simulink library "GTPR_Library"  (R2021a)
settings: Solver=VariableStepAuto  StartTime=0.0  StopTime=10.0  RelTol=1e-3
values from neighbouring files (symbols this model uses):
  aA = 0.5    [SimMechanics_GTPR_OpenLoop_CircularMotion_VS_ClosedLoop.m]
  aB = 0.5    [SimMechanics_GTPR_OpenLoop_CircularMotion_VS_ClosedLoop.m]
  aC = 0.5    [SimMechanics_GTPR_OpenLoop_CircularMotion_VS_ClosedLoop.m]
  alphaAB = deg2rad(120)    [SimMechanics_GTPR_OpenLoop_CircularMotion_VS_ClosedLoop.m]
  alphaAC = deg2rad(240)    [SimMechanics_GTPR_OpenLoop_CircularMotion_VS_ClosedLoop.m]
  eA = 0.28    [SimMechanics_GTPR_OpenLoop_CircularMotion_VS_ClosedLoop.m]
  eB = 0.28    [SimMechanics_GTPR_OpenLoop_CircularMotion_VS_ClosedLoop.m]
  eC = 0.28    [SimMechanics_GTPR_OpenLoop_CircularMotion_VS_ClosedLoop.m]
  g = -9.81    [SimMechanics_GTPR_OpenLoop_CircularMotion_VS_ClosedLoop.m]
  ILA = zeros(3)    [SimMechanics_GTPR_OpenLoop_CircularMotion_VS_ClosedLoop.m]
  IlA = zeros(3)    [SimMechanics_GTPR_OpenLoop_CircularMotion_VS_ClosedLoop.m]
  ILB = zeros(3)    [SimMechanics_GTPR_OpenLoop_CircularMotion_VS_ClosedLoop.m]
  IlB = zeros(3)    [SimMechanics_GTPR_OpenLoop_CircularMotion_VS_ClosedLoop.m]
  ILC = zeros(3)    [SimMechanics_GTPR_OpenLoop_CircularMotion_VS_ClosedLoop.m]
  IlC = zeros(3)    [SimMechanics_GTPR_OpenLoop_CircularMotion_VS_ClosedLoop.m]
  LA = 0.57    [SimMechanics_GTPR_OpenLoop_CircularMotion_VS_ClosedLoop.m]
  lA = 0.9    [SimMechanics_GTPR_OpenLoop_CircularMotion_VS_ClosedLoop.m]
  LB = 0.57    [SimMechanics_GTPR_OpenLoop_CircularMotion_VS_ClosedLoop.m]
  lB = 0.9    [SimMechanics_GTPR_OpenLoop_CircularMotion_VS_ClosedLoop.m]
  LC = 0.57    [SimMechanics_GTPR_OpenLoop_CircularMotion_VS_ClosedLoop.m]
  lC = 0.9    [SimMechanics_GTPR_OpenLoop_CircularMotion_VS_ClosedLoop.m]
  m_unaccounted = 1e-16    [SimMechanics_GTPR_OpenLoop_CircularMotion_VS_ClosedLoop.m]
  mLA = density_upperArm*VLA    (= 1.4415197891)    [SimMechanics_GTPR_OpenLoop_CircularMotion_VS_ClosedLoop.m]
  mlA = density_LowerArm*VlA    (= 0.190851753706)    [SimMechanics_GTPR_OpenLoop_CircularMotion_VS_ClosedLoop.m]
  mLB = density_upperArm*VLB    (= 1.4415197891)    [SimMechanics_GTPR_OpenLoop_CircularMotion_VS_ClosedLoop.m]
  mlB = density_LowerArm*VlB    (= 0.190851753706)    [SimMechanics_GTPR_OpenLoop_CircularMotion_VS_ClosedLoop.m]
  mLC = density_upperArm*VLC    (= 1.4415197891)    [SimMechanics_GTPR_OpenLoop_CircularMotion_VS_ClosedLoop.m]
  mlC = density_LowerArm*VlC    (= 0.190851753706)    [SimMechanics_GTPR_OpenLoop_CircularMotion_VS_ClosedLoop.m]
  mTCP = density_workTriangle * VTCP    [SimMechanics_GTPR_OpenLoop_CircularMotion_VS_ClosedLoop.m]
undefined symbols (not defined in the file or in its folder): dq1, dq2, dq3, q1, q2, q3, X, Y, Z
libraries: sm_lib x83, $bdroot x31, nesl_utility x24
(part 5 of 8)

== matlab function GTPR_Library/Geometry/Inverse Geometry/normalToPlane2 ==
  data: X1 input; nUnit output size=[3 1]; LX input
function nUnit = normalToPlane(X1, LX)

O = [0;0;0];
            
nUnit = cross(O-X1, X1-[0;0;LX]);
nUnit = nUnit / norm(nUnit);

end

    function data = sphereCircleIntersection(cc, rc, nUnit, cs, rs)

    if size(cc) ~= [3,1] %#ok<BDSCA>
        cc = cc';
    end

    if size(cs) ~= [3,1] %#ok<BDSCA>
        cs = cs';
    end

    if size(nUnit) ~= [3,1] %#ok<BDSCA>
        nUnit = nUnit';
    end

    d = dot(nUnit, cc-cs);

    if abs(d) > rs
        data = [];
        return % no intersection
    end

    cp = cs + d*nUnit;

    rp = sqrt(rs^2 - d^2);

    % now the circle circle intersection can be introduced
    dc = norm(cc - cp);

    h = 0.5 + ((rc^2-rp^2)/(2*dc^2));

    ci = cc + h*(cc-cp);

    ri = sqrt(rc^2 - h^2*dc^2);

    % ni = (cc - cp)/d;

    t = cross(cp-cc,nUnit)/norm(cross(cp-cc,nUnit));

    p0 = cc - t*ri + (cc-ci); % Added part for compensation and ci has been modified to cc in both cases
    p1 = cc + t*ri + (cc-ci);

    data.ci = ci;
    data.p0 = p0;
    data.p1 = p1;

    % hold on;
    % plot3(cc(1), cc(2), cc(3), 'bo');
    % quiver3(cc(1), cc(2), cc(3), nUnit(1), nUnit(2), nUnit(3), 'm')
    % 
    % plot3(cs(1), cs(2), cs(3), 'bs');
    % 
    % plot3(ci(1), ci(2), ci(3), 'ro');
    % plot3(p0(1), p0(2), p0(3), 'rx');
    % plot3(p1(1), p1(2), p1(3), 'r*');

    end

== matlab function GTPR_Library/Geometry/Inverse Geometry/sphereCircleIntersection ==
  data: cc input size=[3 1]; p0 output size=[3 1]; rc input; nUnit input size=[3 1]; cs input size=[3 1]; rs input
function p0 = sphereCircleIntersection(cc, rc, nUnit, cs, rs)
%https://gamedev.stackexchange.com/questions/75756/sphere-sphere-intersection-and-circle-sphere-intersection
    if size(cc) ~= [3,1] %#ok<BDSCA>
        cc = cc';
    end

    if size(cs) ~= [3,1] %#ok<BDSCA>
        cs = cs';
    end

    if size(nUnit) ~= [3,1] %#ok<BDSCA>
        nUnit = nUnit';
    end

    d = dot(nUnit, cc-cs);

    if abs(d) > rs
%         data = [];
        p0 = nan;
        return % no intersection
    end

    cp = cs + d*nUnit;

    rp = sqrt(rs^2 - d^2);

    % now the circle circle intersection can be introduced
    dc = norm(cc - cp);

    h = 0.5 + ((rc^2-rp^2)/(2*dc^2));

    ci = cc + h*(cc-cp);

    ri = sqrt(rc^2 - h^2*dc^2);

    % ni = (cc - cp)/d;

    t = cross(cp-cc,nUnit)/norm(cross(cp-cc,nUnit));

    p0 = cc - t*ri + (cc-ci); % Added part for compensation and ci has been modified to cc in both cases
%     p1 = cc + t*ri + (cc-ci);

%     data.ci = ci;
%     data.p0 = p0;
%     data.p1 = p1;

end

== matlab function GTPR_Library/Geometry/Inverse Geometry/sphereCircleIntersection1 ==
  data: cc input size=[3 1]; p0 output size=[3 1]; rc input; nUnit input size=[3 1]; cs input size=[3 1]; rs input
function p0 = sphereCircleIntersection(cc, rc, nUnit, cs, rs)
%https://gamedev.stackexchange.com/questions/75756/sphere-sphere-intersection-and-circle-sphere-intersection
    if size(cc) ~= [3,1] %#ok<BDSCA>
        cc = cc';
    end

    if size(cs) ~= [3,1] %#ok<BDSCA>
        cs = cs';
    end

    if size(nUnit) ~= [3,1] %#ok<BDSCA>
        nUnit = nUnit';
    end

    d = dot(nUnit, cc-cs);

    if abs(d) > rs
%         data = [];
        p0 = nan;
        return % no intersection
    end

    cp = cs + d*nUnit;

    rp = sqrt(rs^2 - d^2);

    % now the circle circle intersection can be introduced
    dc = norm(cc - cp);

    h = 0.5 + ((rc^2-rp^2)/(2*dc^2));

    ci = cc + h*(cc-cp);

    ri = sqrt(rc^2 - h^2*dc^2);

    % ni = (cc - cp)/d;

    t = cross(cp-cc,nUnit)/norm(cross(cp-cc,nUnit));

    p0 = cc - t*ri + (cc-ci); % Added part for compensation and ci has been modified to cc in both cases
%     p1 = cc + t*ri + (cc-ci);

%     data.ci = ci;
%     data.p0 = p0;
%     data.p1 = p1;

end

== matlab function GTPR_Library/Geometry/Inverse Geometry/sphereCircleIntersection2 ==
  data: cc input size=[3 1]; p0 output size=[3 1]; rc input; nUnit input size=[3 1]; cs input size=[3 1]; rs input
function p0 = sphereCircleIntersection(cc, rc, nUnit, cs, rs)
%https://gamedev.stackexchange.com/questions/75756/sphere-sphere-intersection-and-circle-sphere-intersection
    if size(cc) ~= [3,1] %#ok<BDSCA>
        cc = cc';
    end

    if size(cs) ~= [3,1] %#ok<BDSCA>
        cs = cs';
    end

    if size(nUnit) ~= [3,1] %#ok<BDSCA>
        nUnit = nUnit';
    end

    d = dot(nUnit, cc-cs);

    if abs(d) > rs
%         data = [];
        p0 = nan;
        return % no intersection
    end

    cp = cs + d*nUnit;

    rp = sqrt(rs^2 - d^2);

    % now the circle circle intersection can be introduced
    dc = norm(cc - cp);

    h = 0.5 + ((rc^2-rp^2)/(2*dc^2));

    ci = cc + h*(cc-cp);

    ri = sqrt(rc^2 - h^2*dc^2);

    % ni = (cc - cp)/d;

    t = cross(cp-cc,nUnit)/norm(cross(cp-cc,nUnit));

    p0 = cc - t*ri + (cc-ci); % Added part for compensation and ci has been modified to cc in both cases
%     p1 = cc + t*ri + (cc-ci);

%     data.ci = ci;
%     data.p0 = p0;
%     data.p1 = p1;

end

== matlab function GTPR_Library/Other Functions/Inverse Half-Tangent ==
  data: X1 input; q output; X2 input
function q = invHalfTangent(X1, X2)
O = [0;0;0];
OX1 = O-X1;
X2X1 = X2-X1;

q = pi - acos(dot(X2X1,OX1)/(norm(OX1)*norm(X2X1)));

== matlab function GTPR_Library/Geometry/Inverse Geometry/Inverse Half-Tangent ==
  data: X1 input; q output; X2 input
function q = invHalfTangent(X1, X2)
O = [0;0;0];
OX1 = O-X1;
X2X1 = X2-X1;

q = pi - acos(dot(X2X1,OX1)/(norm(OX1)*norm(X2X1)));

== matlab function GTPR_Library/Geometry/Inverse Geometry/Inverse Half-Tangent1 ==
  data: X1 input; q output; X2 input
function q = invHalfTangent(X1, X2)
O = [0;0;0];
OX1 = O-X1;
X2X1 = X2-X1;

q = pi - acos(dot(X2X1,OX1)/(norm(OX1)*norm(X2X1)));

== matlab function GTPR_Library/Geometry/Inverse Geometry/Inverse Half-Tangent2 ==
  data: X1 input; q output; X2 input
function q = invHalfTangent(X1, X2)
O = [0;0;0];
OX1 = O-X1;
X2X1 = X2-X1;

q = pi - acos(dot(X2X1,OX1)/(norm(OX1)*norm(X2X1)));

== matlab function GTPR_Library/Other Functions/Unit Screw [w,v] ==
  data: P2 input; S output; P1 input
function S = fcn(P2,P1)

S = zeros(6,1);

P1P2 = P2-P1;

S(1:3) = P1P2/norm(P1P2);

S(4:6) = cross(P2P1, S(1:3));

== matlab function GTPR_Library/Other Functions/Arm X Screws ==
  data: X1 input; S01X output; X2 input; X3 input; S12X output; S23X output; S34X output; S45X output; S56X output; SLX output; SlX output
function [S01X, S12X, S23X, S34X, S45X, S56X, SLX, SlX] = calculateScrews_ArmX(X1, X2, X3)

    Rz = @(theta)([cos(theta), -sin(theta), 0; sin(theta), cos(theta), 0; 0,0,1]);
    % Getting the Screws of the system:
    % Arm A:
    
    S01X = ones(6,1);
    S12X = ones(6,1);
    S23X = ones(6,1);
    S34X = ones(6,1);
    S45X = ones(6,1);
    S56X = ones(6,1);

    S12X(1:3) = Rz(pi/2) * ((X1)/norm(X1));
    S23X(1:3) = S12X(1:3);
    S34X(1:3) = cross(S23X(1:3),(X3-X2)); 
    S34X(1:3) = S34X(1:3)/norm(S34X(1:3));
    S45X(1:3) = S23X(1:3);
    S56X(1:3) = S34X(1:3);

    S12X(4:6) = cross(X1, S12X(1:3));
    S23X(4:6) = cross(X2, S23X(1:3));
    S34X(4:6) = cross(X2, S34X(1:3));
    S45X(4:6) = cross(X3, S45X(1:3));
    S56X(4:6) = cross(X3, S56X(1:3));

    obj.S01A = zeros(6,1);

    % Reciprocal Screws (lower arms, passive joints):
    SlX = ones(6,1);
    SlX(1:3) = (X3-X2) / norm(X3-X2);
    SlX(4:6) = cross(X3, SlX(1:3));

    % Screws of upper arms:
    SLX = ones(6,1);
    SLX(1:3) = (X2-X1)/(norm(X2-X1));
    SLX(4:6) = cross(X2,SLX(1:3));

== matlab function GTPR_Library/Kinematics/Calculate Jacobian/Arm X Screws ==
  data: X1 input size=[3 1]; S01X output size=[6 1]; X2 input size=[3 1]; X3 input size=[3 1]; S12X output size=[6 1]; S23X output size=[6 1]; S34X output size=[6 1]; S45X output size=[6 1]; S56X output size=[6 1]; SLX output size=[6 1]; SlX output size=[6 1]
function [S01X, S12X, S23X, S34X, S45X, S56X, SLX, SlX] = calculateScrews_ArmX(X1, X2, X3)

    Rz = @(theta)([cos(theta), -sin(theta), 0; sin(theta), cos(theta), 0; 0,0,1]);
    % Getting the Screws of the system:
    % Arm A:
    
    S01X = ones(6,1);
    S12X = ones(6,1);
    S23X = ones(6,1);
    S34X = ones(6,1);
    S45X = ones(6,1);
    S56X = ones(6,1);

    S12X(1:3) = Rz(pi/2) * ((X1)/norm(X1));
    S23X(1:3) = S12X(1:3);
    S34X(1:3) = cross(S23X(1:3),(X3-X2)); 
    S34X(1:3) = S34X(1:3)/norm(S34X(1:3));
    S45X(1:3) = S23X(1:3);
    S56X(1:3) = S34X(1:3);

    S12X(4:6) = cross(X1, S12X(1:3));
    S23X(4:6) = cross(X2, S23X(1:3));
    S34X(4:6) = cross(X2, S34X(1:3));
    S45X(4:6) = cross(X3, S45X(1:3));
    S56X(4:6) = cross(X3, S56X(1:3));

    obj.S01A = zeros(6,1);

    % Reciprocal Screws (lower arms, passive joints):
    SlX = ones(6,1);
    SlX(1:3) = (X3-X2) / norm(X3-X2);
    SlX(4:6) = cross(X3, SlX(1:3));

    % Screws of upper arms:
    SLX = ones(6,1);
    SLX(1:3) = (X2-X1)/(norm(X2-X1));
    SLX(4:6) = cross(X2,SLX(1:3));

== matlab function GTPR_Library/Kinematics/Calculate Jacobian/Arm X Screws1 ==
  data: X1 input size=[3 1]; S01X output size=[6 1]; X2 input size=[3 1]; X3 input size=[3 1]; S12X output size=[6 1]; S23X output size=[6 1]; S34X output size=[6 1]; S45X output size=[6 1]; S56X output size=[6 1]; SLX output size=[6 1]; SlX output size=[6 1]
function [S01X, S12X, S23X, S34X, S45X, S56X, SLX, SlX] = calculateScrews_ArmX(X1, X2, X3)

    Rz = @(theta)([cos(theta), -sin(theta), 0; sin(theta), cos(theta), 0; 0,0,1]);
    % Getting the Screws of the system:
    % Arm A:
    
    S01X = ones(6,1);
    S12X = ones(6,1);
    S23X = ones(6,1);
    S34X = ones(6,1);
    S45X = ones(6,1);
    S56X = ones(6,1);

    S12X(1:3) = Rz(pi/2) * ((X1)/norm(X1));
    S23X(1:3) = S12X(1:3);
    S34X(1:3) = cross(S23X(1:3),(X3-X2)); 
    S34X(1:3) = S34X(1:3)/norm(S34X(1:3));
    S45X(1:3) = S23X(1:3);
    S56X(1:3) = S34X(1:3);

    S12X(4:6) = cross(X1, S12X(1:3));
    S23X(4:6) = cross(X2, S23X(1:3));
    S34X(4:6) = cross(X2, S34X(1:3));
    S45X(4:6) = cross(X3, S45X(1:3));
    S56X(4:6) = cross(X3, S56X(1:3));

    obj.S01A = zeros(6,1);

    % Reciprocal Screws (lower arms, passive joints):
    SlX = ones(6,1);
    SlX(1:3) = (X3-X2) / norm(X3-X2);
    SlX(4:6) = cross(X3, SlX(1:3));

    % Screws of upper arms:
    SLX = ones(6,1);
    SLX(1:3) = (X2-X1)/(norm(X2-X1));
    SLX(4:6) = cross(X2,SLX(1:3));

== matlab function GTPR_Library/Kinematics/Calculate Jacobian/Arm X Screws2 ==
  data: X1 input size=[3 1]; S01X output size=[6 1]; X2 input size=[3 1]; X3 input size=[3 1]; S12X output size=[6 1]; S23X output size=[6 1]; S34X output size=[6 1]; S45X output size=[6 1]; S56X output size=[6 1]; SLX output size=[6 1]; SlX output size=[6 1]
function [S01X, S12X, S23X, S34X, S45X, S56X, SLX, SlX] = calculateScrews_ArmX(X1, X2, X3)

    Rz = @(theta)([cos(theta), -sin(theta), 0; sin(theta), cos(theta), 0; 0,0,1]);
    % Getting the Screws of the system:
    % Arm A:
    
    S01X = ones(6,1);
    S12X = ones(6,1);
    S23X = ones(6,1);
    S34X = ones(6,1);
    S45X = ones(6,1);
    S56X = ones(6,1);

    S12X(1:3) = Rz(pi/2) * ((X1)/norm(X1));
    S23X(1:3) = S12X(1:3);
    S34X(1:3) = cross(S23X(1:3),(X3-X2)); 
    S34X(1:3) = S34X(1:3)/norm(S34X(1:3));
    S45X(1:3) = S23X(1:3);
    S56X(1:3) = S34X(1:3);

    S12X(4:6) = cross(X1, S12X(1:3));
    S23X(4:6) = cross(X2, S23X(1:3));
    S34X(4:6) = cross(X2, S34X(1:3));
    S45X(4:6) = cross(X3, S45X(1:3));
    S56X(4:6) = cross(X3, S56X(1:3));

    obj.S01A = zeros(6,1);

    % Reciprocal Screws (lower arms, passive joints):
    SlX = ones(6,1);
    SlX(1:3) = (X3-X2) / norm(X3-X2);
    SlX(4:6) = cross(X3, SlX(1:3));

    % Screws of upper arms:
    SLX = ones(6,1);
    SLX(1:3) = (X2-X1)/(norm(X2-X1));
    SLX(4:6) = cross(X2,SLX(1:3));

== matlab function GTPR_Library/Other Functions/J_A ==
  data: SlA input; J_A output; SlB input; SlC input
function J_A = Jacobi_part_A(SlA, SlB, SlC)

J_A = [SlA(1:3), SlB(1:3), SlC(1:3)]';

== matlab function GTPR_Library/Other Functions/J_B ==
  data: S12A input; J_B output; S12B input; S12C input; SlA input; SlB input; SlC input
function J_B = Jacobi_part_B(S12A, S12B, S12C, SlA, SlB, SlC)

BB1 = kleinForm(S12A,SlA);
BB2 = kleinForm(S12B,SlB);
BB3 = kleinForm(S12C,SlC);
J_B = diag([BB1, BB2, BB3]);

== matlab function GTPR_Library/Other Functions/Jacobian ==
  data: J_A input; J output; J_B input; J_inv output
function [J, J_inv] = GTPR_Jacobian(J_A, J_B)

J = J_A\J_B;
J_inv = J_B\J_A;

== matlab function GTPR_Library/Kinematics/Calculate Jacobian/cJ_A ==
  data: SlA input; J_A output; SlB input; SlC input
function J_A = Jacobi_part_A(SlA, SlB, SlC)

J_A = [SlA(1:3), SlB(1:3), SlC(1:3)]';

== matlab function GTPR_Library/Kinematics/Calculate Jacobian/cJ_B ==
  data: S12A input; J_B output; S12B input; S12C input; SlA input; SlB input; SlC input
function J_B = Jacobi_part_B(S12A, S12B, S12C, SlA, SlB, SlC)

BB1 = kleinForm(S12A,SlA);
BB2 = kleinForm(S12B,SlB);
BB3 = kleinForm(S12C,SlC);
J_B = diag([BB1, BB2, BB3]);

== matlab function GTPR_Library/Kinematics/Calculate Jacobian/Jacobian ==
  data: J_A input; J output; J_B input; J_inv output
function [J, J_inv] = GTPR_Jacobian(J_A, J_B)

J = J_A\J_B;
J_inv = J_B\J_A;

== matlab function GTPR_Library/Kinematics/Direct Kinematics Acceleration/directKinematics_Acceleration ==
  data: ddq input; a output; J_A input; J_B input; J_C input
function a = directKinematics_Acceleration(ddq, J_A, J_B, J_C)

    a = J_A\(J_B*ddq + J_C);

== matlab function GTPR_Library/Kinematics/Direct Kinematics Acceleration/Jacobian_C ==
  data: ScrewsArm_A input; J_C output; ScrewsArm_B input; ScrewsArm_C input
function J_C = Jacobian_C(ScrewsArm_A,ScrewsArm_B,ScrewsArm_C)
    S01A = ScrewsArm_A.S01A;
    S12A = ScrewsArm_A.S12A;
    S23A = ScrewsArm_A.S23A;
    S34A = ScrewsArm_A.S34A;
    S45A = ScrewsArm_A.S45A;
    S56A = ScrewsArm_A.S56A;
    
    S01B = ScrewsArm_B.S01B;
    S12B = ScrewsArm_B.S12B;
    S23B = ScrewsArm_B.S23B;
    S34B = ScrewsArm_B.S34B;
    S45B = ScrewsArm_B.S45B;
    S56B = ScrewsArm_B.S56B;

    S01C = ScrewsArm_C.S01C;
    S12C = ScrewsArm_C.S12C;
    S23C = ScrewsArm_C.S23C;
    S34C = ScrewsArm_C.S34C;
    S45C = ScrewsArm_C.S45C;
    S56C = ScrewsArm_C.S56C;
    
    SlA = ScrewsArm_A.SlA;
    SlB = ScrewsArm_A.SlB;
    SlC = ScrewsArm_A.SlC;

    LieA = lieProduct(phiA(1)*S01A, phiA(2)*S12A + phiA(3)*S23A + phiA(4)*S34A + phiA(5)*S45A + phiA(6)*S56A) + ... 
               lieProduct(phiA(2)*S12A, phiA(3)*S23A + phiA(4)*S34A + phiA(5)*S45A + phiA(6)*S56A) + ...
               lieProduct(phiA(3)*S23A, phiA(4)*S34A + phiA(5)*S45A + phiA(6)*S56A) + ...
               lieProduct(phiA(4)*S34A, phiA(5)*S45A + phiA(6)*S56A) + ...
               lieProduct(phiA(5)*S45A, phiA(6)*S56A);

    LieB = lieProduct(phiB(1)*S01B, phiB(2)*S12B + phiB(3)*S23B + phiB(4)*S34B + phiB(5)*S45B + phiB(6)*S56B) + ... 
               lieProduct(phiB(2)*S12B, phiB(3)*S23B + phiB(4)*S34B + phiB(5)*S45B + phiB(6)*S56B) + ...
               lieProduct(phiB(3)*S23B, phiB(4)*S34B + phiB(5)*S45B + phiB(6)*S56B) + ...
               lieProduct(phiB(4)*S34B, phiB(5)*S45B + phiB(6)*S56B) + ...
               lieProduct(phiB(5)*S45B, phiB(6)*S56B);

    LieC = lieProduct(phiC(1)*S01C, phiC(2)*S12C + phiC(3)*S23C + phiC(4)*S34C + phiC(5)*S45C + phiC(6)*S56C) + ... 
               lieProduct(phiC(2)*S12C, phiC(3)*S23C + phiC(4)*S34C + phiC(5)*S45C + phiC(6)*S56C) + ...
               lieProduct(phiC(3)*S23C, phiC(4)*S34C + phiC(5)*S45C + phiC(6)*S56C) + ...
               lieProduct(phiC(4)*S34C, phiC(5)*S45C + phiC(6)*S56C) + ...
               lieProduct(phiC(5)*S45C, phiC(6)*S56C);

    J_C = [kleinForm(LieA, SlA); kleinForm(LieB, SlB); kleinForm(LieC, SlC)];

== matlab function GTPR_Library/Kinematics/Inverse Kinematics Acceleration/Jacobian_C ==
  data: ScrewsArm_A input; J_C output; ScrewsArm_B input; ScrewsArm_C input; v input
function J_C = Jacobian_C(ScrewsArm_A,ScrewsArm_B,ScrewsArm_C, v)
    S01A = ScrewsArm_A.S01;
    S12A = ScrewsArm_A.S12;
    S23A = ScrewsArm_A.S23;
    S34A = ScrewsArm_A.S34;
    S45A = ScrewsArm_A.S45;
    S56A = ScrewsArm_A.S56;
    
    S01B = ScrewsArm_B.S01;
    S12B = ScrewsArm_B.S12;
    S23B = ScrewsArm_B.S23;
    S34B = ScrewsArm_B.S34;
    S45B = ScrewsArm_B.S45;
    S56B = ScrewsArm_B.S56;

    S01C = ScrewsArm_C.S01;
    S12C = ScrewsArm_C.S12;
    S23C = ScrewsArm_C.S23;
    S34C = ScrewsArm_C.S34;
    S45C = ScrewsArm_C.S45;
    S56C = ScrewsArm_C.S56;
    
    SlA = ScrewsArm_A.Sl;
    SlB = ScrewsArm_A.Sl;
    SlC = ScrewsArm_A.Sl;

    V = [0;0;0;v];
    
    J_armA = [ones(6,1), S12A, S23A, S34A, S45A, S56A];
    J_armB = [ones(6,1), S12B, S23B, S34B, S45B, S56B];
    J_armC = [ones(6,1), S12C, S23C, S34C, S45C, S56C];

    phiA = J_armA\V;
    phiB = J_armB\V;
    phiC = J_armC\V;
    
    
    LieA = lieProduct(phiA(1)*S01A, phiA(2)*S12A + phiA(3)*S23A + phiA(4)*S34A + phiA(5)*S45A + phiA(6)*S56A) + ... 
               lieProduct(phiA(2)*S12A, phiA(3)*S23A + phiA(4)*S34A + phiA(5)*S45A + phiA(6)*S56A) + ...
               lieProduct(phiA(3)*S23A, phiA(4)*S34A + phiA(5)*S45A + phiA(6)*S56A) + ...
               lieProduct(phiA(4)*S34A, phiA(5)*S45A + phiA(6)*S56A) + ...
               lieProduct(phiA(5)*S45A, phiA(6)*S56A);

    LieB = lieProduct(phiB(1)*S01B, phiB(2)*S12B + phiB(3)*S23B + phiB(4)*S34B + phiB(5)*S45B + phiB(6)*S56B) + ... 
               lieProduct(phiB(2)*S12B, phiB(3)*S23B + phiB(4)*S34B + phiB(5)*S45B + phiB(6)*S56B) + ...
               lieProduct(phiB(3)*S23B, phiB(4)*S34B + phiB(5)*S45B + phiB(6)*S56B) + ...
               lieProduct(phiB(4)*S34B, phiB(5)*S45B + phiB(6)*S56B) + ...
               lieProduct(phiB(5)*S45B, phiB(6)*S56B);

    LieC = lieProduct(phiC(1)*S01C, phiC(2)*S12C + phiC(3)*S23C + phiC(4)*S34C + phiC(5)*S45C + phiC(6)*S56C) + ... 
               lieProduct(phiC(2)*S12C, phiC(3)*S23C + phiC(4)*S34C + phiC(5)*S45C + phiC(6)*S56C) + ...
               lieProduct(phiC(3)*S23C, phiC(4)*S34C + phiC(5)*S45C + phiC(6)*S56C) + ...
               lieProduct(phiC(4)*S34C, phiC(5)*S45C + phiC(6)*S56C) + ...
               lieProduct(phiC(5)*S45C, phiC(6)*S56C);

    J_C = [kleinForm(LieA, SlA); kleinForm(LieB, SlB); kleinForm(LieC, SlC)];

    
function out = lieProduct(S1,S2)
   out = zeros(6,1);
   out(1:3) = cross(S1(1:3), S2(1:3));
   out(4:6) = cross(S1(1:3),S2(4:6)) - cross(S2(1:3), S1(4:6));
end

end

== matlab function GTPR_Library/Kinematics/Inverse Kinematics Acceleration/inverseKinematics_Acceleration ==
  data: a input; ddq output; J_A input; J_B input; J_C input
function ddq = directKinematics_Acceleration(a, J_A, J_B, J_C)

    ddq = J_B\(J_A*a - J_C);

== matlab function GTPR_Library/Dynamics/Initialize Dynamic Equations/If Action Subsystem/Initialize Dynamics ==
  data: filepath input
function InitDynamics(filepath)

data = fileread(filepath);
eval(data);

== matlab function GTPR_Library/Dynamics/Inverse Dynamics/lambdas ==
  data: M_dGammadxyz input; lambda output; Mxyz input; Fext input
function lambda = lambdas(M_dGammadxyz, Mxyz, Fext)

lambda = M_dGammadxyz\(Mxyz - Fext);

== matlab function GTPR_Library/Dynamics/Inverse Dynamics/tauCalc ==
  data: tau output; Mddq input; lambda input; dGammaAdq1 input; dGammaBdq2 input; dGammaCdq3 input
function tau = tauCalc(Mddq, lambda, dGammaAdq1, dGammaBdq2, dGammaCdq3)

tau = Mddq - lambda.*[dGammaAdq1; dGammaBdq2; dGammaCdq3];

== matlab function GTPR_Library/Dynamics/Inverse Dynamics/Mxyz/MATLAB Function ==
  data: Mat input; I11 output; I12 output; I13 output; I21 output; I22 output; I23 output; I31 output; I32 output; I33 output
function [I11, I12, I13, I21, I22, I23, I31, I32, I33] = MatrixToElements(Mat)

I11 = Mat(1,1);
I12 = Mat(1,2);
I13 = Mat(1,3);

I21 = Mat(2,1);
I22 = Mat(2,2);
I23 = Mat(2,3);

I31 = Mat(3,1);
I32 = Mat(3,2);
I33 = Mat(3,3);

== matlab function GTPR_Library/Dynamics/Inverse Dynamics/Mddq/MATLAB Function1 ==
  data: Mat input; I11 output; I12 output; I13 output; I21 output; I22 output; I23 output; I31 output; I32 output; I33 output
function [I11, I12, I13, I21, I22, I23, I31, I32, I33] = MatrixToElements(Mat)

I11 = Mat(1,1);
I12 = Mat(1,2);
I13 = Mat(1,3);

I21 = Mat(2,1);
I22 = Mat(2,2);
I23 = Mat(2,3);

I31 = Mat(3,1);
I32 = Mat(3,2);
I33 = Mat(3,3);

== matlab function GTPR_Library/Dynamics/Inverse Dynamics/Mddq/MATLAB Function2 ==
  data: Mat input; I11 output; I12 output; I13 output; I21 output; I22 output; I23 output; I31 output; I32 output; I33 output
function [I11, I12, I13, I21, I22, I23, I31, I32, I33] = MatrixToElements(Mat)

I11 = Mat(1,1);
I12 = Mat(1,2);
I13 = Mat(1,3);

I21 = Mat(2,1);
I22 = Mat(2,2);
I23 = Mat(2,3);

I31 = Mat(3,1);
I32 = Mat(3,2);
I33 = Mat(3,3);

== matlab function GTPR_Library/Dynamics/Inverse Dynamics/Mddq/MATLAB Function3 ==
  data: Mat input; I11 output; I12 output; I13 output; I21 output; I22 output; I23 output; I31 output; I32 output; I33 output
function [I11, I12, I13, I21, I22, I23, I31, I32, I33] = MatrixToElements(Mat)

I11 = Mat(1,1);
I12 = Mat(1,2);
I13 = Mat(1,3);

I21 = Mat(2,1);
I22 = Mat(2,2);
I23 = Mat(2,3);

I31 = Mat(3,1);
I32 = Mat(3,2);
I33 = Mat(3,3);

== matlab function GTPR_Library/Dynamics/Inverse Dynamics/Mddq/MATLAB Function4 ==
  data: Mat input; I11 output; I12 output; I13 output; I21 output; I22 output; I23 output; I31 output; I32 output; I33 output
function [I11, I12, I13, I21, I22, I23, I31, I32, I33] = MatrixToElements(Mat)

I11 = Mat(1,1);
I12 = Mat(1,2);
I13 = Mat(1,3);

I21 = Mat(2,1);
I22 = Mat(2,2);
I23 = Mat(2,3);

I31 = Mat(3,1);
I32 = Mat(3,2);
I33 = Mat(3,3);

== matlab function GTPR_Library/Dynamics/Inverse Dynamics/Mddq/MATLAB Function5 ==
  data: Mat input; I11 output; I12 output; I13 output; I21 output; I22 output; I23 output; I31 output; I32 output; I33 output
function [I11, I12, I13, I21, I22, I23, I31, I32, I33] = MatrixToElements(Mat)

I11 = Mat(1,1);
I12 = Mat(1,2);
I13 = Mat(1,3);

I21 = Mat(2,1);
I22 = Mat(2,2);
I23 = Mat(2,3);

I31 = Mat(3,1);
I32 = Mat(3,2);
I33 = Mat(3,3);

== matlab function GTPR_Library/Dynamics/Inverse Dynamics/Mddq/MATLAB Function6 ==
  data: Mat input; I11 output; I12 output; I13 output; I21 output; I22 output; I23 output; I31 output; I32 output; I33 output
function [I11, I12, I13, I21, I22, I23, I31, I32, I33] = MatrixToElements(Mat)

I11 = Mat(1,1);
I12 = Mat(1,2);
I13 = Mat(1,3);

I21 = Mat(2,1);
I22 = Mat(2,2);
I23 = Mat(2,3);

I31 = Mat(3,1);
I32 = Mat(3,2);
I33 = Mat(3,3);

== matlab function GTPR_Library/Dynamics/Inverse Dynamics/Mxyz/MATLAB Function1 ==
  data: Mat input; I11 output; I12 output; I13 output; I21 output; I22 output; I23 output; I31 output; I32 output; I33 output
function [I11, I12, I13, I21, I22, I23, I31, I32, I33] = MatrixToElements(Mat)

I11 = Mat(1,1);
I12 = Mat(1,2);
I13 = Mat(1,3);

I21 = Mat(2,1);
I22 = Mat(2,2);
I23 = Mat(2,3);

I31 = Mat(3,1);
I32 = Mat(3,2);
I33 = Mat(3,3);

== matlab function GTPR_Library/Dynamics/Inverse Dynamics/Mxyz/MATLAB Function2 ==
  data: Mat input; I11 output; I12 output; I13 output; I21 output; I22 output; I23 output; I31 output; I32 output; I33 output
function [I11, I12, I13, I21, I22, I23, I31, I32, I33] = MatrixToElements(Mat)

I11 = Mat(1,1);
I12 = Mat(1,2);
I13 = Mat(1,3);

I21 = Mat(2,1);
I22 = Mat(2,2);
I23 = Mat(2,3);

I31 = Mat(3,1);
I32 = Mat(3,2);
I33 = Mat(3,3);

== matlab function GTPR_Library/Kinematics/Calculate Jacobian/MATLAB Function ==
  data: S01 input size=[6 1]; S output Bus: ScrewBus; S12 input size=[6 1]; S23 input size=[6 1]; S34 input size=[6 1]; S45 input size=[6 1]; S56 input size=[6 1]; SL input size=[6 1]; Sl input size=[6 1]
function S = makeScrewSystemForArm(S01, S12, S23, S34, S45, S56, SL, Sl)

S.S01 = S01;
S.S12 = S12;
S.S23 = S23;
S.S34 = S34;
S.S45 = S45;
S.S56 = S56;
S.SL = SL;
S.Sl = Sl;

== matlab function GTPR_Library/Kinematics/Calculate Jacobian/MATLAB Function1 ==
  data: S01 input; S output Bus: ScrewBus; S12 input; S23 input; S34 input; S45 input; S56 input; SL input; Sl input
function S = makeScrewSystemForArm(S01, S12, S23, S34, S45, S56, SL, Sl)

S.S01 = S01;
S.S12 = S12;
S.S23 = S23;
S.S34 = S34;
S.S45 = S45;
S.S56 = S56;
S.SL = SL;
S.Sl = Sl;

== matlab function GTPR_Library/Kinematics/Calculate Jacobian/MATLAB Function2 ==
  data: S01 input size=[6 1]; S output Bus: ScrewBus; S12 input size=[6 1]; S23 input size=[6 1]; S34 input size=[6 1]; S45 input size=[6 1]; S56 input size=[6 1]; SL input size=[6 1]; Sl input size=[6 1]
function S = makeScrewSystemForArm(S01, S12, S23, S34, S45, S56, SL, Sl)

S.S01 = S01;
S.S12 = S12;
S.S23 = S23;
S.S34 = S34;
S.S45 = S45;
S.S56 = S56;
S.SL = SL;
S.Sl = Sl;
